simulink library "BMS_MAIN_LIB"  (R2023b)
settings: Solver=VariableStepAuto  StartTime=0.0  StopTime=10.0  RelTol=1e-3
undefined symbols (not defined in the file): SAMPLE_TIME_100MS
libraries: simulink x1
settings Model: Creator=Somashekar M  LastModifiedBy=Somashekar M

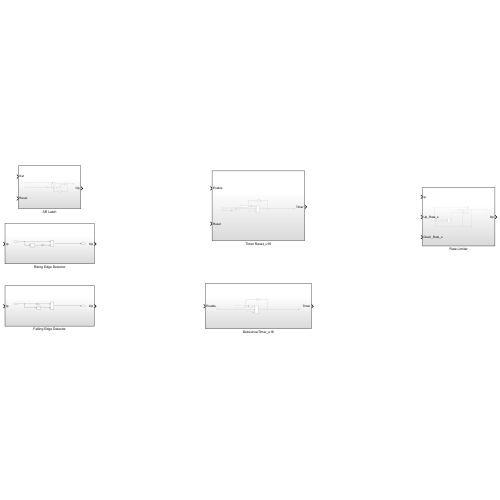
[thumbnail: Simulink's stored preview of the top-level diagram]
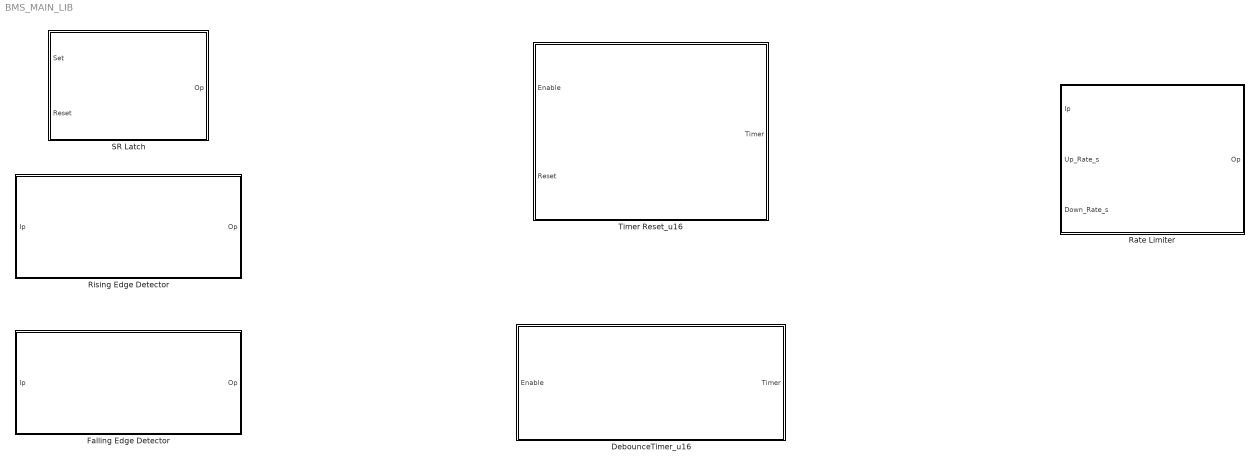
== system BMS_MAIN_LIB ==
  DebounceTimer_u16 : Subsystem
  Falling Edge Detector : Subsystem
  Rate Limiter : Subsystem
  Rising Edge Detector : Subsystem
  SR Latch : Subsystem
  Timer Reset_u16 : Subsystem

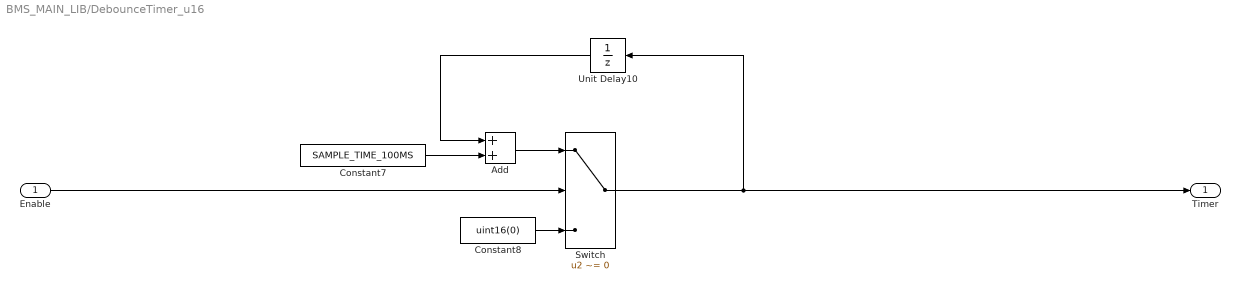
== system BMS_MAIN_LIB/DebounceTimer_u16 ==
  Enable : Inport
  Add : Sum
  Constant7 : Constant  Value=SAMPLE_TIME_100MS
  Constant8 : Constant  Value=uint16(0)
  Switch : Switch  Criteria=u2 ~= 0  SaturateOnIntegerOverflow=off  InputSameDT=off
  Unit Delay10 : UnitDelay  SampleTime=-1  HasFrameUpgradeWarning=on
  Timer : Outport
  wires:
  Add/1 -> Switch/1
  Constant7/1 -> Add/2
  Enable/1 -> Switch/2
  Unit Delay10/1 -> Add/1
  Constant8/1 -> Switch/3
  Switch/1 -> Timer/1, Unit Delay10/1

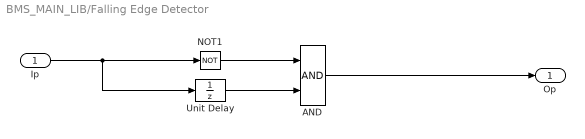
== system BMS_MAIN_LIB/Falling Edge Detector ==
  Ip : Inport
  AND : Logic  AllPortsSameDT=off  OutDataTypeStr=boolean
  NOT1 : Logic  Operator=NOT  IconShape=distinctive  AllPortsSameDT=off  OutDataTypeStr=boolean
  Unit Delay : UnitDelay  SampleTime=-1  HasFrameUpgradeWarning=on
  Op : Outport
  wires:
  Unit Delay/1 -> AND/2
  AND/1 -> Op/1
  Ip/1 -> NOT1/1, Unit Delay/1
  NOT1/1 -> AND/1

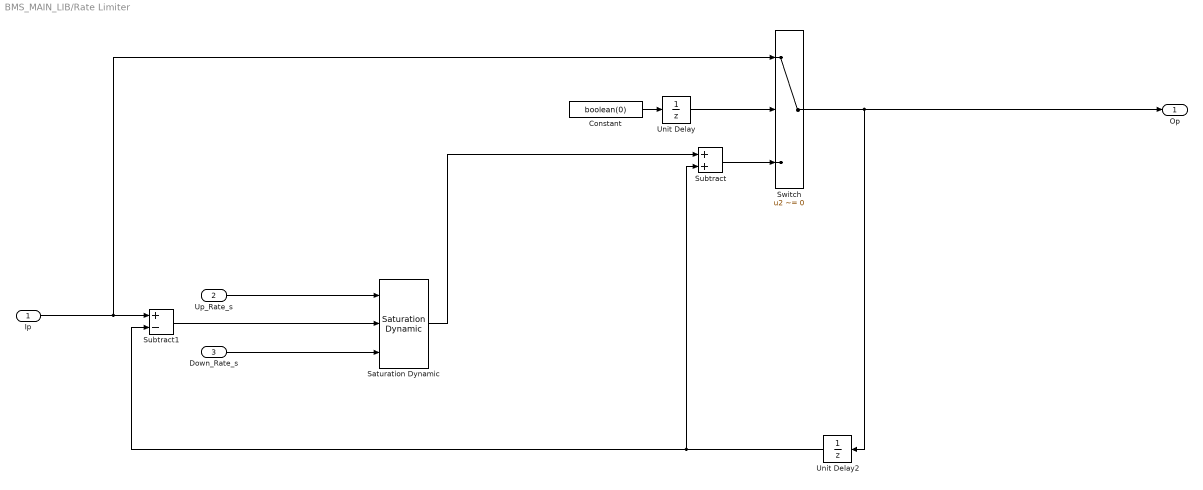
== system BMS_MAIN_LIB/Rate Limiter ==
  Ip : Inport
  Up_Rate_s : Inport  Port=2
  Down_Rate_s : Inport  Port=3
  Constant : Constant  Value=boolean(0)
  Saturation Dynamic : simulink/Discontinuities/Saturation Dynamic  OutMin=[]  OutMax=[]  OutDataTypeStr=Inherit: Same as second input  OutDataType=fixdt(1, 16)  OutScaling=2^-10  DoSatur=off
  Subtract : Sum
  Subtract1 : Sum  Inputs=+-
  Switch : Switch  Criteria=u2 ~= 0  SaturateOnIntegerOverflow=off  InputSameDT=off
  Unit Delay : UnitDelay  InitialCondition=boolean(1)  SampleTime=-1  HasFrameUpgradeWarning=on
  Unit Delay2 : UnitDelay  SampleTime=-1  HasFrameUpgradeWarning=on
  Op : Outport
  wires:
  Subtract/1 -> Switch/3
  Unit Delay/1 -> Switch/2
  Constant/1 -> Unit Delay/1
  Ip/1 -> Switch/1, Subtract1/1
  Down_Rate_s/1 -> Saturation Dynamic/3
  Unit Delay2/1 -> Subtract/2, Subtract1/2
  Subtract1/1 -> Saturation Dynamic/2
  Saturation Dynamic/1 -> Subtract/1
  Switch/1 -> Op/1, Unit Delay2/1
  Up_Rate_s/1 -> Saturation Dynamic/1

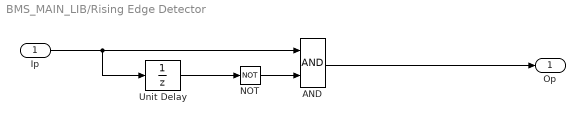
== system BMS_MAIN_LIB/Rising Edge Detector ==
  Ip : Inport
  AND : Logic  AllPortsSameDT=off  OutDataTypeStr=boolean
  NOT : Logic  Operator=NOT  IconShape=distinctive  AllPortsSameDT=off  OutDataTypeStr=boolean
  Unit Delay : UnitDelay  SampleTime=-1  HasFrameUpgradeWarning=on
  Op : Outport
  wires:
  Ip/1 -> Unit Delay/1, AND/1
  AND/1 -> Op/1
  NOT/1 -> AND/2
  Unit Delay/1 -> NOT/1

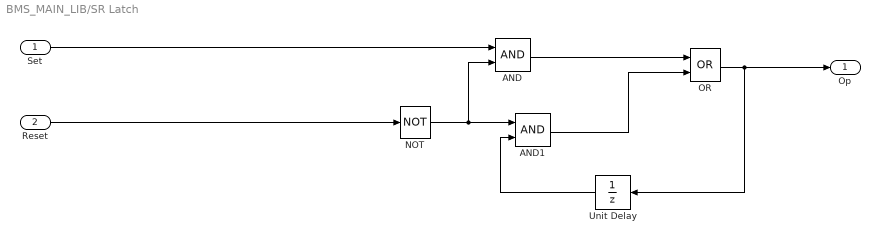
== system BMS_MAIN_LIB/SR Latch ==
  Set : Inport
  Reset : Inport  Port=2
  AND : Logic  AllPortsSameDT=off  OutDataTypeStr=boolean
  AND1 : Logic  AllPortsSameDT=off  OutDataTypeStr=boolean
  NOT : Logic  Operator=NOT  IconShape=distinctive  AllPortsSameDT=off  OutDataTypeStr=boolean
  OR : Logic  Operator=OR  AllPortsSameDT=off  OutDataTypeStr=boolean
  Unit Delay : UnitDelay  SampleTime=-1  HasFrameUpgradeWarning=on
  Op : Outport
  wires:
  Unit Delay/1 -> AND1/2
  Set/1 -> AND/1
  AND1/1 -> OR/2
  NOT/1 -> AND1/1, AND/2
  OR/1 -> Unit Delay/1, Op/1
  AND/1 -> OR/1
  Reset/1 -> NOT/1

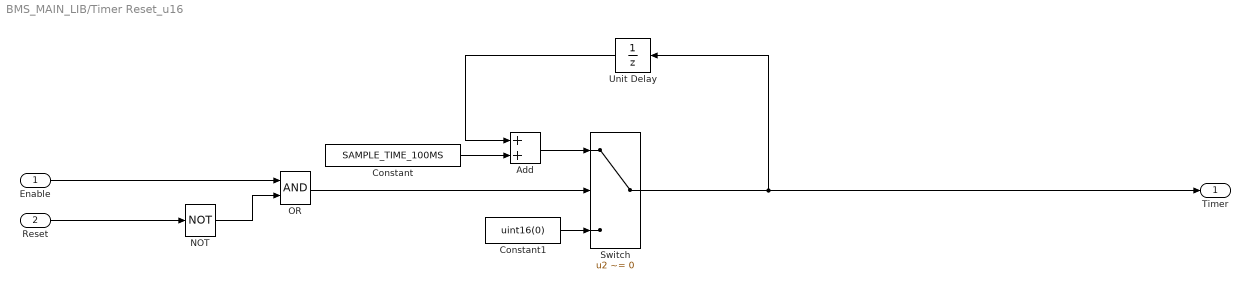
== system BMS_MAIN_LIB/Timer Reset_u16 ==
  Enable : Inport
  Reset : Inport  Port=2
  Add : Sum
  Constant : Constant  Value=SAMPLE_TIME_100MS  OutDataTypeStr=uint16
  Constant1 : Constant  Value=uint16(0)
  NOT : Logic  Operator=NOT  IconShape=distinctive  AllPortsSameDT=off  OutDataTypeStr=boolean
  OR : Logic  AllPortsSameDT=off  OutDataTypeStr=boolean
  Switch : Switch  Criteria=u2 ~= 0  SaturateOnIntegerOverflow=off  InputSameDT=off
  Unit Delay : UnitDelay  SampleTime=-1  HasFrameUpgradeWarning=on
  Timer : Outport
  wires:
  Enable/1 -> OR/1
  Switch/1 -> Timer/1, Unit Delay/1
  Unit Delay/1 -> Add/1
  Constant/1 -> Add/2
  Add/1 -> Switch/1
  Constant1/1 -> Switch/3
  Reset/1 -> NOT/1
  NOT/1 -> OR/2
  OR/1 -> Switch/2
